simulink model "diagsteer_blocks"  (Simulink 6.1)
settings: Solver=FixedStepDiscrete  StartTime=round(t(1)*10000)/10000  StopTime=36000  FixedStep=round((t(2)-t(1))*10000)/10000  RelTol=1e-3
values from neighbouring files (symbols this model uses):
  Ts = 0.002    [DSC_Control_Analysis.m]    (also in DSC_Control_Analysis_Exp.m; DSC_Speed_Control_Analysis.m; EC_params_nissan.m; Ext_MPCPara.m = SSD.Ts)
undefined symbols (not defined in the file or in its folder): Lkal_left, Lkal_right, Lkal_yaw, param, sglu
settings Model: Creator=cgadda  LastModifiedBy=Shad Laws  ExtModeAutoUpdateStatusClock=off
settings DataIOCC: SaveOutput=off  SignalLogging=off  SaveTime=off  SignalLoggingName=sigsOut
settings HardwareCC: TargetUnknown=on
settings GRTTargetCC: ModelReferenceCompliant=off  MatFileLogging=off

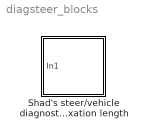
== system diagsteer_blocks ==
  Shad's steer/vehicle diagnostic w/ relaxation length : Subsystem  AncestorBlock=|  mask{paramfile=p1_params, sglufile=nissan_steer_lookup_data, kalfile=diagsteerkalmancalc, outname=outs1, tunev=15.5, tunel=0, tuner=0}
      | offline_estimators/Shad's steer//vehicle diagnostic
      | w// relaxation length
      mask prompts: paramfile "Vehicle params filename"; sglufile "Steer lookups filename"; kalfile "Kalman gains filename"; outname "Output variable name"; tunev "Tuning velocity"; tunel "Tuning left angle"; tuner "Tuning right angle"
      mask init:
      | eval(strrep(paramfile,'.m',''));
      | eval(strrep(sglufile,'.m',''));
      | eval(['[Lkal_yaw,Lkal_left,Lkal_right]=' strrep(kalfile,'.m','') '(param,sglu,' tunev ',' tunel ',' tuner ');']);
      | set_param([gcb '/Output'],'VariableName',outname);
      mask Display: disp(outname);

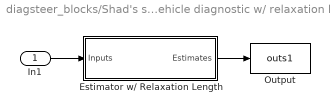
== system diagsteer_blocks/Shad's steer/vehicle diagnostic w/ relaxation length ==
  In1 : Inport  Port=1  LatchInput=off
  Estimator w/ Relaxation Length : Subsystem
  Output : ToWorkspace  VariableName=outs1  SampleTime=-1  SaveFormat=Array
  wires:
  Estimator w/ Relaxation Length/1(Estimates) -> Output/1
  In1/1 -> Estimator w/ Relaxation Length/1(Inputs)

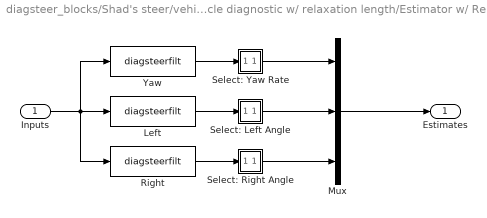
== system diagsteer_blocks/Shad's steer/vehicle diagnostic w/ relaxation length/Estimator w/ Relaxation Length ==
  Inputs : Inport  Port=1  LatchInput=off
  Left : S-Function  FunctionName=diagsteerfilt  Parameters=Ts,param,sglu,Lkal_left
  Mux : Mux  Inputs=3
  Right : S-Function  FunctionName=diagsteerfilt  Parameters=Ts,param,sglu,Lkal_right
  Select: Left Angle : Subsystem  mask{indices=2, width=3}
      mask prompts: indices "Signal indices"; width "Input width"
      mask init:
      | ic=length(indices);
      | 
      | K=zeros(ic,width);
      | 
      | for ii=1:ic,
      | 	K(ii,indices(ii))=1;
      | end
      mask Display: disp(indices)
  Select: Right Angle : Subsystem  mask{indices=3, width=3}
      mask prompts: indices "Signal indices"; width "Input width"
      mask init:
      | ic=length(indices);
      | 
      | K=zeros(ic,width);
      | 
      | for ii=1:ic,
      | 	K(ii,indices(ii))=1;
      | end
      mask Display: disp(indices)
  Select: Yaw Rate : Subsystem  mask{indices=1, width=3}
      mask prompts: indices "Signal indices"; width "Input width"
      mask init:
      | ic=length(indices);
      | 
      | K=zeros(ic,width);
      | 
      | for ii=1:ic,
      | 	K(ii,indices(ii))=1;
      | end
      mask Display: disp(indices)
  Yaw : S-Function  FunctionName=diagsteerfilt  Parameters=Ts,param,sglu,Lkal_yaw
  Estimates : Outport
  wires:
  Mux/1 -> Estimates/1
  Select: Right Angle/1(Out1) -> Mux/3
  Select: Left Angle/1(Out1) -> Mux/2
  Select: Yaw Rate/1(Out1) -> Mux/1
  Inputs/1 -> Right/1, Yaw/1, Left/1
  Right/1 -> Select: Right Angle/1(In1)
  Left/1 -> Select: Left Angle/1(In1)
  Yaw/1 -> Select: Yaw Rate/1(In1)

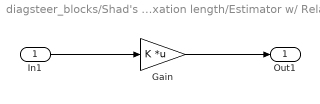
== system diagsteer_blocks/Shad's steer/vehicle diagnostic w/ relaxation length/Estimator w/ Relaxation Length/Select: Left Angle ==
  In1 : Inport  Port=1  LatchInput=off
  Gain : Gain  Gain=K  Multiplication=Matrix(K*u)  SaturateOnIntegerOverflow=on
  Out1 : Outport
  wires:
  In1/1 -> Gain/1
  Gain/1 -> Out1/1

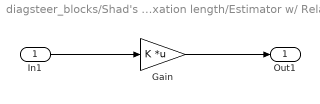
== system diagsteer_blocks/Shad's steer/vehicle diagnostic w/ relaxation length/Estimator w/ Relaxation Length/Select: Right Angle ==
  In1 : Inport  Port=1  LatchInput=off
  Gain : Gain  Gain=K  Multiplication=Matrix(K*u)  SaturateOnIntegerOverflow=on
  Out1 : Outport
  wires:
  In1/1 -> Gain/1
  Gain/1 -> Out1/1

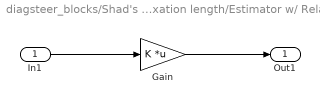
== system diagsteer_blocks/Shad's steer/vehicle diagnostic w/ relaxation length/Estimator w/ Relaxation Length/Select: Yaw Rate ==
  In1 : Inport  Port=1  LatchInput=off
  Gain : Gain  Gain=K  Multiplication=Matrix(K*u)  SaturateOnIntegerOverflow=on
  Out1 : Outport
  wires:
  In1/1 -> Gain/1
  Gain/1 -> Out1/1
